simulink model "Transient_analysis_model"  (R2019b)
settings: Solver=VariableStepAuto  StartTime=0.0  StopTime=10.0  RelTol=1e-3
settings Model: Creator=DELL  LastModifiedBy=DELL

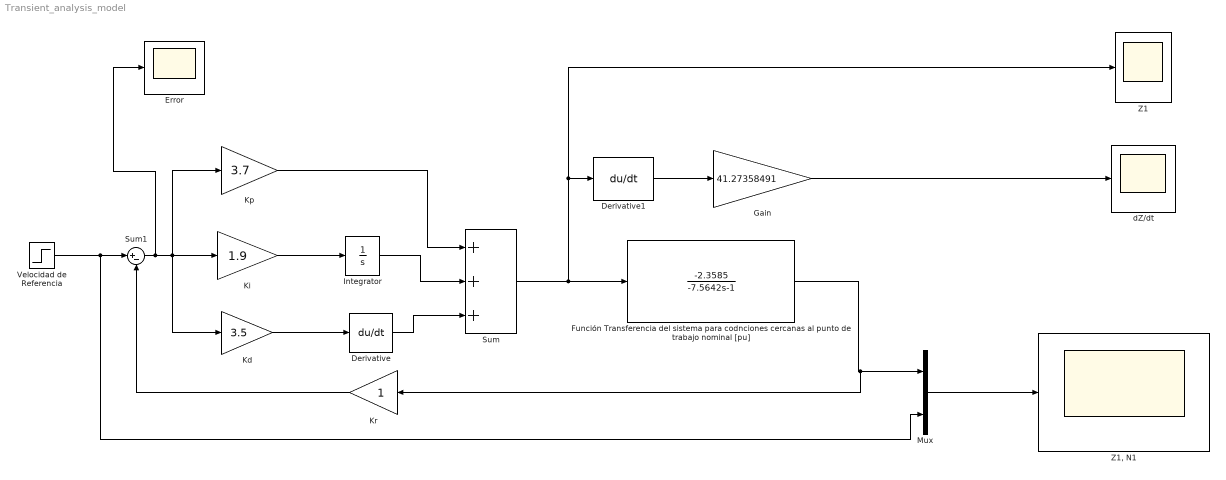
== system Transient_analysis_model ==
  Derivative : Derivative
  Derivative1 : Derivative
  Error : Scope
  Función Transferencia del sistema para codnciones cercanas al punto de trabajo nominal [pu] : TransferFcn  Numerator=-2.3585  Denominator=[-7.5642 -1]
  Gain : Gain  Gain=41.27358491
  Integrator : Integrator
  Kd : Gain  Gain=3.5
  Ki : Gain  Gain=1.9
  Kp : Gain  Gain=3.7
  Kr : Gain
  Mux : Mux  Inputs=2
  Sum : Sum  Inputs=+++
  Sum1 : Sum  Inputs=|+-
  Velocidad de Referencia : Step  Time=0  SampleTime=0
  Z1 : Scope
  "Z1, N1" : Scope
  dZ/dt : Scope
  wires:
  Velocidad de Referencia/1 -> Mux/2, Sum1/1
  Sum1/1 -> Error/1, Kp/1, Ki/1, Kd/1
  Ki/1 -> Integrator/1
  Integrator/1 -> Sum/2
  Kr/1 -> Sum1/2
  Kp/1 -> Sum/1
  Kd/1 -> Derivative/1
  Derivative/1 -> Sum/3
  Sum/1 -> Función Transferencia del sistema para codnciones cercanas al punto de trabajo nominal [pu]/1, Derivative1/1, Z1/1
  Derivative1/1 -> Gain/1
  Función Transferencia del sistema para codnciones cercanas al punto de trabajo nominal [pu]/1 -> Kr/1, Mux/1
  Mux/1 -> "Z1, N1"/1
  Gain/1 -> dZ/dt/1
